simulink model "autovalori_sim"  (R2022b)
settings: Solver=VariableStepAuto  StartTime=0.0  StopTime=10  RelTol=1e-3
values from neighbouring files (symbols this model uses):
  A = [-0.051 0 -0.144 -0.056 0 0 0 0 0 0 0 0 ... (169 elements, 13x13)]    [Elicottero.mat]
  B = [0 0 0 0 0 0 0.68 3.043 0 0 0 0 ... (52 elements, 13x4)]    [Elicottero.mat]
undefined symbols (not defined in the file or in its folder): Aobs, Bobs, C, Cobs, D, Dobs, K_i, K_s, x0_obs
settings Model: Creator=valen  LastModifiedBy=valen
settings ModelReferenceCC: EnableRefExpFcnMdlSchedulingChecks=on

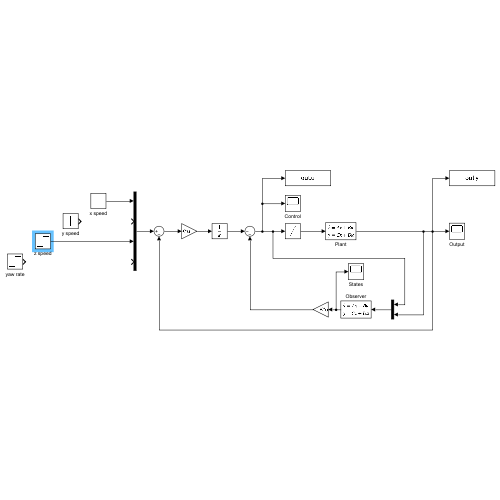
[thumbnail: Simulink's stored preview of the top-level diagram]
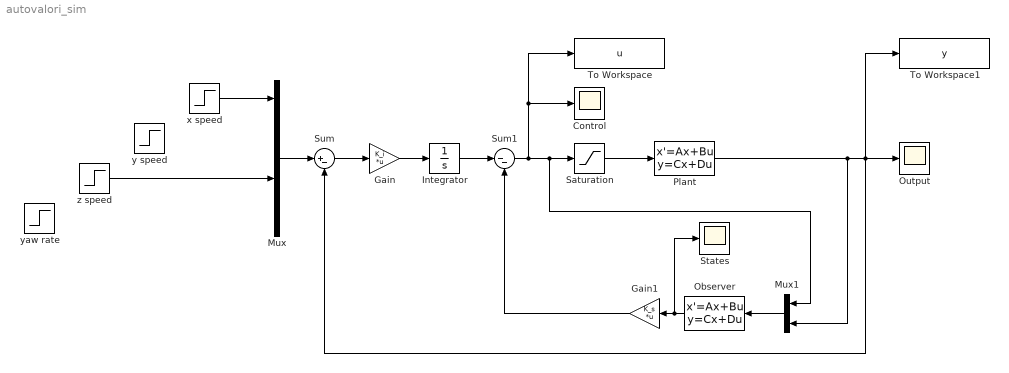
== system autovalori_sim ==
  Control : Scope
  Gain : Gain  Gain=K_i  Multiplication=Matrix(K*u)
  Gain1 : Gain  Gain=K_s  Multiplication=Matrix(K*u)
  Integrator : Integrator
  Mux : Mux
  Mux1 : Mux  Inputs=2
  Observer : StateSpace  A=Aobs  B=Bobs  C=Cobs  D=Dobs  InitialCondition=x0_obs
  Output : Scope
  Plant : StateSpace  A=A  B=B  C=C  D=D  InitialCondition=0
  Saturation : Saturate  UpperLimit=1  LowerLimit=-1
  States : Scope
  Sum : Sum  Inputs=|+-
  Sum1 : Sum  Inputs=|--
  To Workspace : ToWorkspace  VariableName=u  SaveFormat=Structure With Time  SampleTime=-1
  To Workspace1 : ToWorkspace  VariableName=y  SaveFormat=Structure With Time  SampleTime=-1
  x speed : Step  Time=0  SampleTime=0
  y speed : Step  Time=0  SampleTime=0
  yaw rate : Step  Time=0  SampleTime=0
  z speed : Step  Time=5  After=0.5  SampleTime=0
  wires:
  Integrator/1 -> Sum1/1
  Sum1/1 -> To Workspace/1, Control/1, Saturation/1, Mux1/1
  Mux1/1 -> Observer/1
  Observer/1 -> States/1, Gain1/1
  Gain1/1 -> Sum1/2
  Mux/1 -> Sum/1
  Gain/1 -> Integrator/1
  Sum/1 -> Gain/1
  Plant/1 -> Mux1/2, To Workspace1/1, Output/1, Sum/2
  Saturation/1 -> Plant/1
  z speed/1 -> Mux/3
  x speed/1 -> Mux/1
